simulink model "Main"  (R2017b)
settings: Solver=VariableStepAuto  StartTime=0.0  StopTime=10.0  RelTol=1e-3
values from neighbouring files (symbols this model uses):
  cp = 3    [Task1c.m]    (also in Task2.m = 0.4; Task3.m = 0.4; Task4.m = 0.4; Task6.m = 0.8)
  hd = hd_mat(i)    [Task2.m]    (also in Task3.m; task5.m = mp*(2*w*z+a))
  hi = hi_mat    (= 0)    [Task2.m]    (also in Task3.m = hi_mat(k); task5.m = a*w^2)
  hp = hp_mat(j)    [Task2.m]    (also in Task3.m; task5.m = w^2+2*w*a*z-kp)
  kp = 6.32    [Task1c.m]    (also in Task2.m; Task3.m; Task4.m; Task6.m)
  mp = 0.16    [Task1c.m]    (also in Task2.m; Task3.m; Task4.m; Task6.m)
  src = 1    [H_inf_ctrl.m]    (also in Task2.m = 2; Task3.m = 3; Task6.m = 3; Task8.m)
undefined symbols (not defined in the file or in its folder): sigbuilder_block
libraries: simulink x1
settings Model: Creator=Dell  LastModifiedBy=Dell

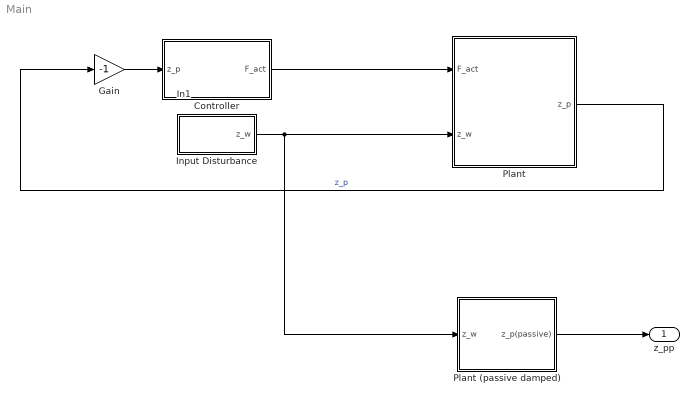
== system Main ==
  In1 : Inport
  Controller : Subsystem
  Gain : Gain  Gain=-1
  Input Disturbance : Subsystem
  Plant : Subsystem
  Plant (passive damped) : Subsystem
  z_pp : Outport
  wires:
  Controller/1(F_act) -> Plant/1(F_act)
  Gain/1 -> Controller/1(z_p)
  Plant/1(z_p) -> Gain/1  "z_p"
  Input Disturbance/1(z_w) -> Plant (passive damped)/1(z_w), Plant/2(z_w)
  Plant (passive damped)/1(z_p(passive)) -> z_pp/1

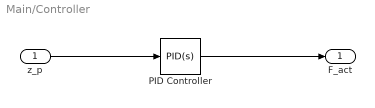
== system Main/Controller ==
  z_p : Inport
  PID Controller : simulink/Continuous/PID Controller  Controller=PID  TimeDomain=Continuous-time  SampleTime=-1  IntegratorMethod=Forward Euler  FilterMethod=Forward Euler  Form=Parallel  UseFilter=on  ControllerParametersSource=internal  P=hp  I=hi  D=hd  N=100  InitialConditionSource=internal  InitialConditionForIntegrator=0  InitialConditionForFilter=0  ExternalReset=none  LimitOutput=off  UpperSaturationLimit=inf  LowerSaturationLimit=-inf  LinearizeAsGain=on  AntiWindupMode=none  Kb=1  TrackingMode=off  Kt=1  PParamMin=[]  PParamMax=[]  IParamMin=[]  IParamMax=[]  DParamMin=[]  DParamMax=[]  NParamMin=[]  NParamMax=[]  KbParamMin=[]  KbParamMax=[]  KtParamMin=[]  KtParamMax=[]  POutMin=[]  POutMax=[]  IOutMin=[]  IOutMax=[]  DOutMin=[]  DOutMax=[]  NOutMin=[]  NOutMax=[]  KbOutMin=[]  KbOutMax=[]  KtOutMin=[]  KtOutMax=[]  IntegratorOutMin=[]  IntegratorOutMax=[]  FilterOutMin=[]  FilterOutMax=[]  SumOutMin=[]  SumOutMax=[]  SumI1OutMin=[]  SumI1OutMax=[]  SumI2OutMin=[]  SumI2OutMax=[]  SumI3OutMin=[]  SumI3OutMax=[]  SumDOutMin=[]  SumDOutMax=[]  SaturationOutMin=[]  SaturationOutMax=[]  IntegratorContinuousStateAttributes=''  IntegratorStateMustResolveToSignalObject=off  IntegratorRTWStateStorageClass=Auto  FilterContinuousStateAttributes=''  FilterStateMustResolveToSignalObject=off  FilterRTWStateStorageClass=Auto  DifferentiatorICPrevScaledInput=0  DifferentiatorOutMin=[]  DifferentiatorOutMax=[]  InitialConditionSetting=State (most efficient)  FilterDiffOutCoefMin=[]  FilterDiffOutCoefMax=[]  SumDenOutMin=[]  SumDenOutMax=[]  SumNumOutMin=[]  SumNumOutMax=[]  ReciprocalOutMin=[]  ReciprocalOutMax=[]  DivideOutMin=[]  DivideOutMax=[]  TunerSelectOption=Transfer Function Based (PID Tuner App)
  F_act : Outport
  wires:
  z_p/1 -> PID Controller/1
  PID Controller/1 -> F_act/1

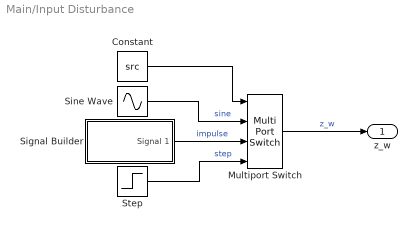
== system Main/Input Disturbance ==
  Constant : Constant  Value=src
  Multiport Switch : MultiPortSwitch
  Signal Builder : Subsystem  Tag=STV Subsys  LoadFcn=sigbuilder_block('load');  StartFcn=sigbuilder_block('start');  StopFcn=sigbuilder_block('stop');  ClipboardFcn=sigbuilder_block('clipboard');  mask(Sigbuilder block){tuvar=[0:10]}
      mask help: Simulink:masks:SigbuilderBlock_MD
      mask init:
      | if ~strcmp(get_param(bdroot(gcbh),'SimulationStatus'),'stopped') tuvar = sigbuilder_block('maskInit'); end
      settings: CopyFcn=sigbuilder_block('copy');  DeleteFcn=sigbuilder_block('delete');  ModelCloseFcn=sigbuilder_block('modelClose');  PreSaveFcn=sigbuilder_block('preSave');  PauseFcn=sigbuilder_block('pause');  ContinueFcn=sigbuilder_block('continue');  NameChangeFcn=sigbuilder_block('namechange');  OpenFcn=sigbuilder_block('open',[437.6 199.2 550.4 400 ]);  CloseFcn=sigbuilder_block('close');
      mask Display: plot(0, 0, 100, 100,[2, 2, 32, 32, 2], [68, 8, 8, 68, 68],[32, 2], [38, 38], [32, 19, 2],[53, 60, 44], [32, 17, 17, 2],[16, 16, 31, 31]);txt = getActiveGroup(gcbh);text(2, 100, txt,'verticalAlignment', 'top');
  Sine Wave : Sin  Amplitude=0.05  Frequency=5  SampleTime=0
  Step : Step  Time=0  SampleTime=0
  z_w : Outport
  wires:
  Sine Wave/1 -> Multiport Switch/2  "sine"
  Signal Builder/1(Signal 1) -> Multiport Switch/3  "impulse"
  Multiport Switch/1 -> z_w/1  "z_w"
  Step/1 -> Multiport Switch/4  "step"
  Constant/1 -> Multiport Switch/1

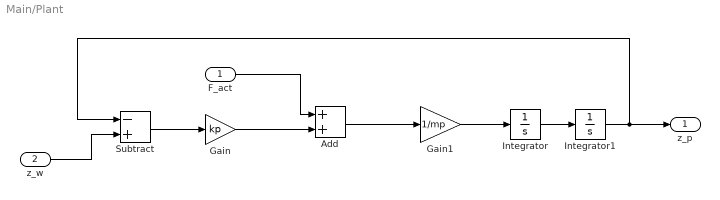
== system Main/Plant ==
  F_act : Inport
  z_w : Inport  Port=2
  Add : Sum
  Gain : Gain  Gain=kp
  Gain1 : Gain  Gain=1/mp
  Integrator : Integrator
  Integrator1 : Integrator
  Subtract : Sum  Inputs=-+
  z_p : Outport
  wires:
  z_w/1 -> Subtract/2
  Subtract/1 -> Gain/1
  F_act/1 -> Add/1
  Gain/1 -> Add/2
  Add/1 -> Gain1/1
  Gain1/1 -> Integrator/1
  Integrator/1 -> Integrator1/1
  Integrator1/1 -> z_p/1, Subtract/1

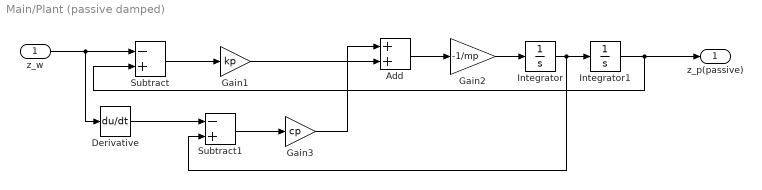
== system Main/Plant (passive damped) ==
  z_w : Inport
  Add : Sum
  Derivative : Derivative
  Gain1 : Gain  Gain=kp
  Gain2 : Gain  Gain=-1/mp
  Gain3 : Gain  Gain=cp
  Integrator : Integrator
  Integrator1 : Integrator
  Subtract : Sum  Inputs=-+
  Subtract1 : Sum  Inputs=-+
  z_p(passive) : Outport
  wires:
  z_w/1 -> Subtract/1, Derivative/1
  Subtract1/1 -> Gain3/1
  Derivative/1 -> Subtract1/1
  Gain2/1 -> Integrator/1
  Integrator1/1 -> z_p(passive)/1, Subtract/2
  Gain1/1 -> Add/2
  Gain3/1 -> Add/1
  Integrator/1 -> Subtract1/2, Integrator1/1
  Add/1 -> Gain2/1
  Subtract/1 -> Gain1/1

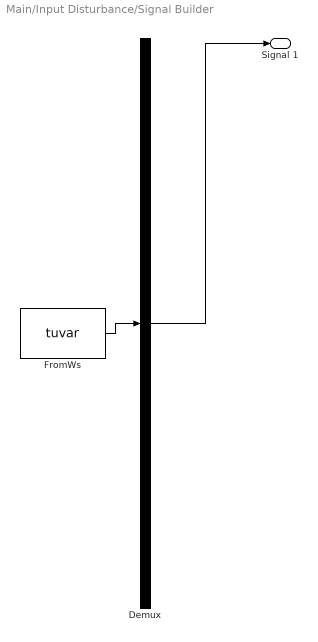
== system Main/Input Disturbance/Signal Builder ==
  Demux : Demux  Tag=STV Demux  Outputs=1
  FromWs : FromWorkspace  Tag=STV FromWs  VariableName=tuvar  SampleTime=0
      SigBuilderData=|
      | common.afterFinalStr = 'Extrapolate'
      | common.sampleTime = 0
      | dataSet.timeRange = [0 10]
      | dataSet.name = 'Group 1'
      | sbobj.Groups.Name = 'Group 1'
      | sbobj.Groups.Signals.Name = 'Signal 1'
      | sbobj.Groups.Signals.XData = [0 2 2 3 3 10]
      | sbobj.Groups.Signals.YData = [0 0 0.05 0.05 0 0]
  Signal 1 : Outport  Tag=STV Outport
  wires:
  Demux/1 -> Signal 1/1
  FromWs/1 -> Demux/1
